simulink model "labp"  (R2023b)
settings: Solver=VariableStepAuto  StartTime=0.0  StopTime=10.0  RelTol=1e-3
undefined symbols (not defined in the file): a, b
libraries: checkpacklib x2
settings Model: Creator=killer  LastModifiedBy=killer

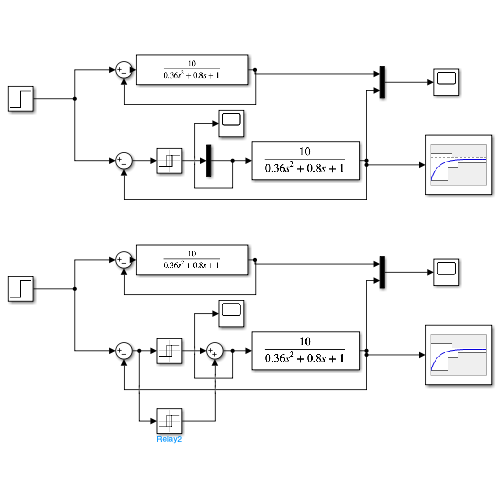
[thumbnail: Simulink's stored preview of the top-level diagram]
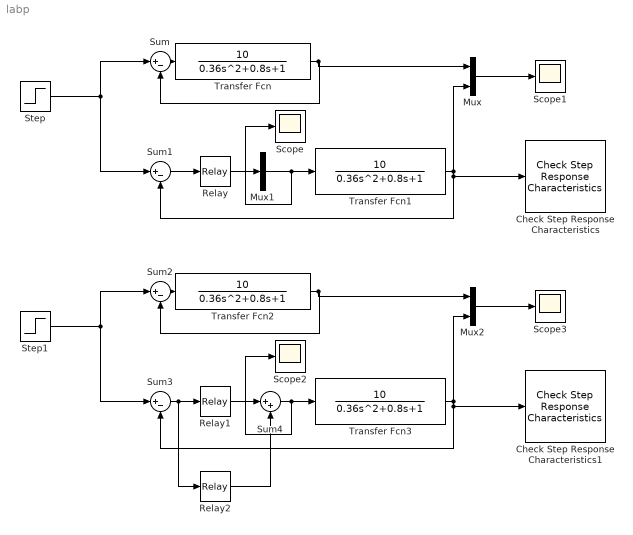
== system labp ==
  Check Step Response Characteristics : checkpacklib/Check Step Response  Characteristics  InstantiateOnLoad=on  enabled=on  stopWhenAssertionFail=off  export=off  ViewDlgPos=[]  OpenViewOnLoad=off  LaunchViewOnOpen=off  TimeUnits=seconds  EnableStepResponseBound=on  InitialValue=0  FinalValue=1  StepTime=0  RiseTime=5  PercentRise=80  SettlingTime=7  PercentSettling=1  PercentOvershoot=10  PercentUndershoot=1
      settings: LibrarySourceBlock=|
      | sdolib/Model Verification/Check Step Response
      | Characteristics
  Check Step Response Characteristics1 : checkpacklib/Check Step Response  Characteristics  InstantiateOnLoad=on  enabled=on  stopWhenAssertionFail=off  export=off  ViewDlgPos=[]  OpenViewOnLoad=off  LaunchViewOnOpen=off  TimeUnits=seconds  EnableStepResponseBound=on  InitialValue=0  FinalValue=1  StepTime=0  RiseTime=5  PercentRise=80  SettlingTime=7  PercentSettling=1  PercentOvershoot=10  PercentUndershoot=1
      settings: LibrarySourceBlock=|
      | sdolib/Model Verification/Check Step Response
      | Characteristics
  Mux : Mux  Inputs=2
  Mux1 : Mux  Inputs=1
  Mux2 : Mux  Inputs=2
  Relay : Relay  OnSwitchValue=a  OffSwitchValue=-a  OnOutputValue=u  OffOutputValue=-u
  Relay1 : Relay  OnSwitchValue=-u  OffSwitchValue=-u-b  OnOutputValue=0  OffOutputValue=-a
  Relay2 : Relay  OnSwitchValue=u+b  OffSwitchValue=u  OnOutputValue=a
  Scope{,1..3} (4 alike) : Scope
  Step : Step  Time=0  SampleTime=0
  Step1 : Step  Time=0  SampleTime=0
  Sum{,1..3} (4 alike) : Sum  Inputs=|+-
  Sum4 : Sum  Inputs=|++
  Transfer Fcn{,1..3} (4 alike) : TransferFcn  Numerator=[10]  Denominator=[0.36 0.8 1]
  wires:
  Mux/1 -> Scope1/1
  Transfer Fcn1/1 -> Sum1/2, Check Step Response Characteristics/1, Mux/2
  Sum/1 -> Transfer Fcn/1
  Transfer Fcn/1 -> Mux/1, Sum/2
  Step/1 -> Sum/1, Sum1/1
  Sum1/1 -> Relay/1
  Relay/1 -> Mux1/1
  Mux1/1 -> Scope/1, Transfer Fcn1/1
  Step1/1 -> Sum2/1, Sum3/1
  Sum4/1 -> Scope2/1, Transfer Fcn3/1
  Transfer Fcn3/1 -> Sum3/2, Check Step Response Characteristics1/1, Mux2/2
  Transfer Fcn2/1 -> Mux2/1, Sum2/2
  Mux2/1 -> Scope3/1
  Sum3/1 -> Relay2/1, Relay1/1
  Sum2/1 -> Transfer Fcn2/1
  Relay1/1 -> Sum4/1
  Relay2/1 -> Sum4/2
